simulink model "AC_DCandDC_AC_Conversion"  (R2024a)
settings: Solver=VariableStepAuto  StartTime=0.0  StopTime=5  RelTol=1e-3
undefined symbols (not defined in the file or in its folder): D1, Delta
libraries: spsSeriesRLCBranchLib x6, spsMosfetLib x6, spsVoltageMeasurementLib x5, spsThreePhaseSeriesRLCBranchLib x3, simulink x3, spsCurrentMeasurementLib x2, spsPiSectionLineLib x2, spsThreePhaseSeriesRLCLoadLib x2, spsThreePhaseTransformerTwoWindingsLib x2, spsThreePhaseVIMeasurementLib x2, spsThreePhaseParallelRLCBranchLib x1, spsSawtoothGeneratorLib x1
settings Model: Creator=Esty  LastModifiedBy=Esty

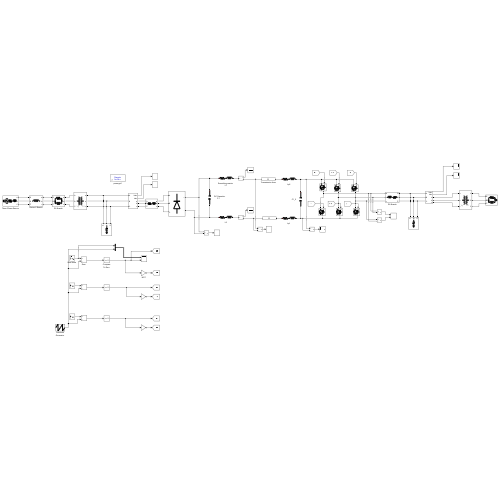
[thumbnail: Simulink's stored preview of the top-level diagram]
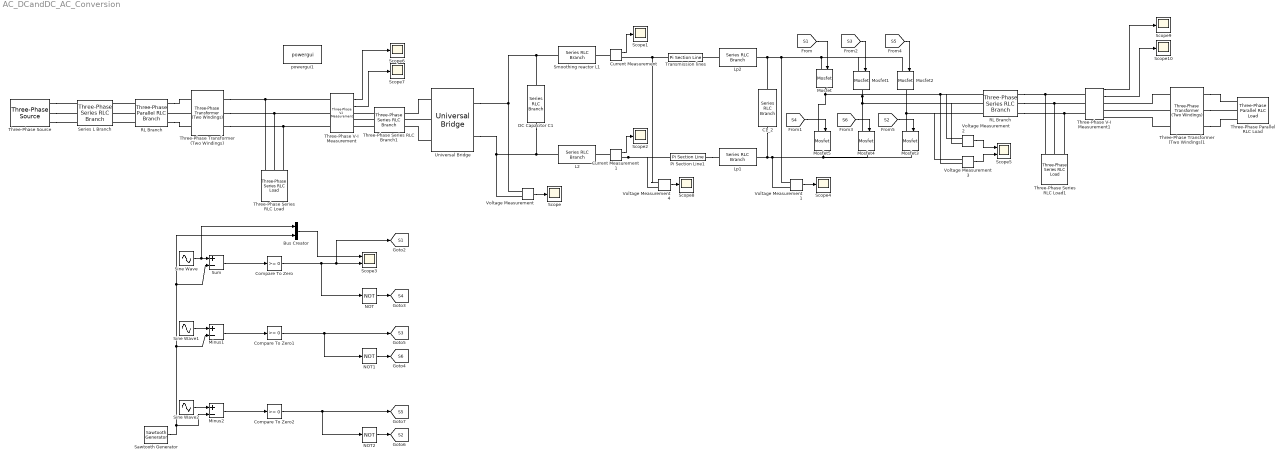
== system AC_DCandDC_AC_Conversion ==
  " RL Branch" : spsThreePhaseSeriesRLCBranchLib/Three-Phase Series RLC Branch  LConnTagsString=A|B|C  RConnTagsString=A|B|C  BranchType=RL  Resistance=0.75  Inductance=0.183  Capacitance=1e-6  Measurements=None
  Bus Creator : BusCreator  Inputs=2
  C1_2 : spsSeriesRLCBranchLib/Series RLC Branch  LConnTagsString=__new0  RConnTagsString=__new0  BranchType=C  Resistance=1  Inductance=1e-3  SetiL0=off  InitialCurrent=0  Capacitance=0.0001  Setx0=off  InitialVoltage=0  Measurements=None
  "Compare To Zero " : simulink/Logic and Bit Operations/Compare To Zero  relop=>=  OutDataTypeStr=boolean
  Compare To Zero1 : simulink/Logic and Bit Operations/Compare To Zero  relop=>=  OutDataTypeStr=boolean
  Compare To Zero2 : simulink/Logic and Bit Operations/Compare To Zero  relop=>=  OutDataTypeStr=boolean
  Current Measurement : spsCurrentMeasurementLib/Current Measurement  PhasorSimulation=off  OutputType=Complex  PSBequivalent=0
  Current Measurement1 : spsCurrentMeasurementLib/Current Measurement  PhasorSimulation=off  OutputType=Complex  PSBequivalent=0
  DC Capacitor C1 : spsSeriesRLCBranchLib/Series RLC Branch  LConnTagsString=__new0  RConnTagsString=__new0  BranchType=C  Resistance=1  Inductance=1e-3  SetiL0=off  InitialCurrent=0  Capacitance=0.005  Setx0=off  InitialVoltage=0  Measurements=None
  L2 : spsSeriesRLCBranchLib/Series RLC Branch  LConnTagsString=__new0  RConnTagsString=__new0  BranchType=RL  Resistance=0.0251  Inductance=1  SetiL0=off  InitialCurrent=0  Capacitance=1e-6  Setx0=off  InitialVoltage=0  Measurements=None
  Lp1 : spsSeriesRLCBranchLib/Series RLC Branch  LConnTagsString=__new0  RConnTagsString=__new0  BranchType=RL  Resistance=0.0251  Inductance=1  SetiL0=off  InitialCurrent=0  Capacitance=1e-6  Setx0=off  InitialVoltage=0  Measurements=None
  Lp2 : spsSeriesRLCBranchLib/Series RLC Branch  LConnTagsString=__new0  RConnTagsString=__new0  BranchType=RL  Resistance=0.0251  Inductance=1  SetiL0=off  InitialCurrent=0  Capacitance=1e-6  Setx0=off  InitialVoltage=0  Measurements=None
  Minus1 : Sum  Inputs=+-
  Minus2 : Sum  Inputs=+-
  Mosfet{,1..5} (6 alike) : spsMosfetLib/Mosfet  Ron=0.1  Lon=0  Rd=0.01  Vfd=0  IC=0  Rs=1e5  Cs=inf  Measurements=off
  "NOT " : Logic  Operator=NOT  IconShape=distinctive  AllPortsSameDT=off  OutDataTypeStr=boolean
  NOT1 : Logic  Operator=NOT  IconShape=distinctive  AllPortsSameDT=off  OutDataTypeStr=boolean
  NOT2 : Logic  Operator=NOT  IconShape=distinctive  AllPortsSameDT=off  OutDataTypeStr=boolean
  Pi Section Line1 : spsPiSectionLineLib/Pi Section Line  LConnTagsString=1  RConnTagsString=1  Phases=1  PiSections=2  Length=75  Frequency=50  Resistance=0.0139  Inductance=0.159e-3  Capacitance=0.23e-6  SpecifyConductance=off  Conductance=0  Measurements=None  Measurements2=None
      settings: LibrarySourceBlock=sps_lib/Power Grid Elements/Pi Section Line
  RL Branch : spsThreePhaseParallelRLCBranchLib/Three-Phase Parallel RLC Branch  LConnTagsString=A|B|C  RConnTagsString=A|B|C  BranchType=RL  Resistance=13.79  Inductance=31.02e-3  Capacitance=1e-6  Measurements=None
  "Sawtooth Generator " : spsSawtoothGeneratorLib/Sawtooth Generator  Freq=5e3  Phase=180  Ts=0
  Scope{,1..2,4,6..10} (9 alike) : Scope
  Scope3 : Scope  NumInputPorts=2
  Scope5 : Scope  NumInputPorts=2
  Series L Branch : spsThreePhaseSeriesRLCBranchLib/Three-Phase Series RLC Branch  LConnTagsString=A|B|C  RConnTagsString=A|B|C  BranchType=L  Resistance=1  Inductance=62.23e-3  Capacitance=1e-6  Measurements=None
  "Sine Wave " : Sin  Frequency=376.99  SampleTime=0
  Sine Wave1 : Sin  Frequency=376.99  Phase=-120*(pi/180)  SampleTime=0
  Sine Wave2 : Sin  Frequency=376.99  Phase=120*(pi/180)  SampleTime=0
  Smoothing reactor L1 : spsSeriesRLCBranchLib/Series RLC Branch  LConnTagsString=__new0  RConnTagsString=__new0  BranchType=RL  Resistance=0.0251  Inductance=1  SetiL0=off  InitialCurrent=0  Capacitance=1e-6  Setx0=off  InitialVoltage=0  Measurements=None
  "Sum " : Sum  Inputs=+-
  Three-Phase Parallel RLC Load : spsThreePhaseParallelRLCLoadLib/Three-Phase Parallel RLC Load  LConnTagsString=A|B|C  Configuration=Y (grounded)  NominalVoltage=230e3  Vabc=[1e3 1e3 1e3]  Vabcp=[1e3 1e3 1e3]  NominalFrequency=50  UnbalancedPower=off  ActivePower=135e3  InductivePower=75e3  CapacitivePower=0  Pabc=[10e3 9e3 11e3]  QLabc=[100 90 110]  QCabc=[100 90 110]  Pabcp=[10e3 9e3 11e3]  QLabcp=[100 90 110]  QCabcp=[100 90 110]  Measurements=None  LoadType=constant Z
  Three-Phase Series RLC Branch1 : spsThreePhaseSeriesRLCBranchLib/Three-Phase Series RLC Branch  LConnTagsString=A|B|C  RConnTagsString=A|B|C  BranchType=RL  Resistance=0.75  Inductance=0.1830  Capacitance=1e-6  Measurements=None
  Three-Phase Series RLC Load : spsThreePhaseSeriesRLCLoadLib/Three-Phase Series RLC Load  LConnTagsString=A|B|C  Configuration=Y (grounded)  NominalVoltage=100e3  Vabc=[1e3 1e3 1e3]  Vabcp=[1e3 1e3 1e3]  NominalFrequency=50  UnbalancedPower=off  ActivePower=0  InductivePower=0  CapacitivePower=200e3  Pabc=[10e3 9e3 11e3]  QLabc=[100 90 110]  QCabc=[100 90 110]  Pabcp=[10e3 9e3 11e3]  QLabcp=[100 90 110]  QCabcp=[100 90 110]  Measurements=None  LoadType=constant Z
  Three-Phase Series RLC Load1 : spsThreePhaseSeriesRLCLoadLib/Three-Phase Series RLC Load  LConnTagsString=A|B|C  Configuration=Y (grounded)  NominalVoltage=100e3  Vabc=[1e3 1e3 1e3]  Vabcp=[1e3 1e3 1e3]  NominalFrequency=50  UnbalancedPower=off  ActivePower=0  InductivePower=0  CapacitivePower=200e3  Pabc=[10e3 9e3 11e3]  QLabc=[100 90 110]  QCabc=[100 90 110]  Pabcp=[10e3 9e3 11e3]  QLabcp=[100 90 110]  QCabcp=[100 90 110]  Measurements=None  LoadType=constant Z
  Three-Phase Transformer (Two Windings) : spsThreePhaseTransformerTwoWindingsLib/Three-Phase Transformer (Two Windings)  Winding1Connection=Yg  Winding2Connection=Delta (D1)  CoreType=Three single-phase transformers  SetSaturation=off  Hysteresis=off  DataFile='hysteresis'  SetInitialFlux=off  Measurements=None  UNITS=pu  NominalPower=[ 200e6 , 50 ]  Winding1=[ 230e3 , 0.0025 , 0.075 ]  Winding2=[ 100e3 , 0.0025 , 0.075 ]  Rm=500  Lm=500  L0=0.5  Saturation=[ 0,0 ; 0.0024,1.2 ; 1.0,1.52 ]  InitialFluxes=[ 0.8 , -0.8 , 0.7 ]  BreakLoop=off  DiscreteSolver=Trapezoidal iterative  DataType=off  TransfoNumber=1
  Three-Phase Transformer (Two Windings)1 : spsThreePhaseTransformerTwoWindingsLib/Three-Phase Transformer (Two Windings)  Winding1Connection=Delta (D1)  Winding2Connection=Yg  CoreType=Three single-phase transformers  SetSaturation=off  Hysteresis=off  DataFile='hysteresis'  SetInitialFlux=off  Measurements=None  UNITS=pu  NominalPower=[ 200e6 , 50 ]  Winding1=[ 230e3*0.88 , 0.0025 , 0.0075 ]  Winding2=[ 100e3 , 0.0025 , 0.075 ]  Rm=500  Lm=500  L0=0.5  Saturation=[ 0,0 ; 0.0024,1.2 ; 1.0,1.52 ]  InitialFluxes=[ 0.8 , -0.8 , 0.7 ]  BreakLoop=off  DiscreteSolver=Trapezoidal iterative  DataType=off  TransfoNumber=1
  Three-Phase V-I Measurement : spsThreePhaseVIMeasurementLib/Three-Phase V-I Measurement  VoltageMeasurement=phase-to-ground  SetLabelV=off  LabelV=Vabc  Vpu=off  VpuLL=off  CurrentMeasurement=yes  SetLabelI=off  LabelI=Iabc  Ipu=off  Pbase=100e6  Vbase=500e3  OutputType=Complex  PhasorSimulation=off  PSBequivalent=0
  Three-Phase V-I Measurement1 : spsThreePhaseVIMeasurementLib/Three-Phase V-I Measurement  VoltageMeasurement=phase-to-ground  SetLabelV=off  LabelV=Vabc  Vpu=off  VpuLL=off  CurrentMeasurement=yes  SetLabelI=off  LabelI=Iabc  Ipu=off  Pbase=100e6  Vbase=500e3  OutputType=Complex  PhasorSimulation=off  PSBequivalent=0
  "Three-Phase Source " : spsThreePhaseSourceLib/Three-Phase Source  InternalConnection=Yg  VoltagePhases=off  Voltage=230e3  PhaseAngle=0  Voltage_phases=[25e3 25e3 25e3]/sqrt(3)  PhaseAngles_phases=[0 -120 +120]  Frequency=50  NonIdealSource=on  SpecifyImpedance=off  Resistance=0.8929  Inductance=16.58e-3  ShortCircuitLevel=100e6  BaseVoltage=25e3  XRratio=7  BusType=swing  Pref=10e3  Qref=0  Prefabc=[10e3, 10e3, 10e3]  Qrefabc=[0, 0, 0]  Qmin=-inf  Qmax=inf
  Transmission lines : spsPiSectionLineLib/Pi Section Line  LConnTagsString=1  RConnTagsString=1  Phases=1  PiSections=2  Length=75  Frequency=50  Resistance=0.0139  Inductance=0.159e-3  Capacitance=0.23e-6  SpecifyConductance=off  Conductance=0  Measurements=None  Measurements2=None
      settings: LibrarySourceBlock=sps_lib/Power Grid Elements/Pi Section Line
  Universal Bridge : spsUniversalBridgeLib/Universal Bridge  Arms=3  SnubberResistance=1e5  SnubberCapacitance=inf  Device=Diodes  Ron=1e-3  Lon=0  ForwardVoltages="[  0  0  ]"  ForwardVoltage=0  GTOparameters=[ 10e-6 , 20e-6 ]  IGBTparameters=[ 1e-6 , 2e-6 ]  Measurements=None  Measurements_2=None  converterType=Rectifier
  Voltage Measurement{,1..4} (5 alike) : spsVoltageMeasurementLib/Voltage Measurement  PhasorSimulation=off  OutputType=Complex  PSBequivalent=0
  powergui1 : sps_lib/powergui  Priority=1  SimulationMode=Discrete  SampleTime=5e-06  frequency=60  Iterations=50  frequencyindice=0  Pbase=100e6  ErrMax=1e-4  UnitsV=kV  UnitsW=MW  buscounter=0  FunctionMessages=off  echomessages=off  EnableUseOfTLC=off  CurrentSourceSwitches=off  DisableSnubberDevices=off  DisableRonSwitches=off  DisableVfSwitches=off  DisplayEquations=off  AutomaticDiscreteSolvers=off  SolverType=Tustin/Backward Euler (TBE)  Interpol=off  ExternalGateDelay=off  methode=off  Ts=100  x0status=blocks  SPID=on  SwTol=0  HookPort=off  NonlinearTolerance=1e-4  nMaxIteration=100  ContinueOnMaxIteration=off  RestoreLinks=warning  ResistiveCurrentMeasurement=off  Frange=[0:2:500]  Ylog=off  Xlog=on  ShowGrid=off  save=off  variable=ZData  structure=0  ZoomFFT=off  StartTime=0.0  cycles=1  DisplayStyle=1  fundamental=60  FreqAxis=off  MaxFrequency=1000  frequencyindicesteady=1  RmsSteady=1  display=off
  tag scope: S1=global, S2=global, S3=global, S4=global, S5=global, S6=global
  wires:
  Voltage Measurement/1 -> Scope/1
  Current Measurement/1 -> Scope1/1
  Current Measurement1/1 -> Scope2/1
  [S4] -> Mosfet5/1
  [S3] -> Mosfet1/1
  [S5] -> Mosfet2/1
  [S2] -> Mosfet3/1
  [S6] -> Mosfet4/1
  Minus2/1 -> Compare To Zero2/1
  "Sum "/1 -> "Compare To Zero "/1
  "Sine Wave "/1 -> Bus Creator/1, "Sum "/1
  Compare To Zero1/1 -> [S3], NOT1/1
  Bus Creator/1 -> Scope3/1
  "NOT "/1 -> [S4]
  Compare To Zero2/1 -> [S5], NOT2/1
  Sine Wave2/1 -> Minus2/1
  "Sawtooth Generator "/1 -> Bus Creator/2, "Sum "/2, Minus1/2, Minus2/2
  NOT2/1 -> [S2]
  Minus1/1 -> Compare To Zero1/1
  "Compare To Zero "/1 -> "NOT "/1, [S1], Scope3/2
  Sine Wave1/1 -> Minus1/1
  NOT1/1 -> [S6]
  [S1] -> Mosfet/1
  Voltage Measurement1/1 -> Scope4/1
  Voltage Measurement2/1 -> Scope5/1
  Voltage Measurement3/1 -> Scope5/2
  Three-Phase V-I Measurement/1 -> Scope6/1
  Three-Phase V-I Measurement/2 -> Scope7/1
  Voltage Measurement4/1 -> Scope8/1
  Three-Phase V-I Measurement1/1 -> Scope9/1
  Three-Phase V-I Measurement1/2 -> Scope10/1
  connections:
  "Three-Phase Source "/RConn1 -- Series L Branch/LConn1
  "Three-Phase Source "/RConn2 -- Series L Branch/LConn2
  "Three-Phase Source "/RConn3 -- Series L Branch/LConn3
  RL Branch/LConn1 -- Series L Branch/RConn1
  RL Branch/LConn2 -- Series L Branch/RConn2
  RL Branch/LConn3 -- Series L Branch/RConn3
  Three-Phase Transformer (Two Windings)/LConn2 -- RL Branch/RConn2
  RL Branch/RConn1 -- Three-Phase Transformer (Two Windings)/LConn1
  RL Branch/RConn3 -- Three-Phase Transformer (Two Windings)/LConn3
  Three-Phase Transformer (Two Windings)/RConn1 -- Three-Phase Series RLC Load/LConn1 -- Three-Phase V-I Measurement/LConn1
  Three-Phase Transformer (Two Windings)/RConn2 -- Three-Phase V-I Measurement/LConn2 -- Three-Phase Series RLC Load/LConn2
  Three-Phase Transformer (Two Windings)/RConn3 -- Three-Phase V-I Measurement/LConn3 -- Three-Phase Series RLC Load/LConn3
  Universal Bridge/LConn1 -- Three-Phase Series RLC Branch1/RConn1
  Universal Bridge/LConn2 -- Three-Phase Series RLC Branch1/RConn2
  Universal Bridge/LConn3 -- Three-Phase Series RLC Branch1/RConn3
  Universal Bridge/RConn1 -- DC Capacitor C1/LConn1 -- Smoothing reactor L1/LConn1 -- Voltage Measurement/LConn1
  Current Measurement1/LConn1 -- L2/RConn1
  Current Measurement/LConn1 -- Smoothing reactor L1/RConn1
  Universal Bridge/RConn2 -- Voltage Measurement/LConn2 -- DC Capacitor C1/RConn1 -- L2/LConn1
  Transmission lines/LConn1 -- Voltage Measurement4/LConn1 -- Current Measurement/RConn1
  Current Measurement1/RConn1 -- Pi Section Line1/LConn1 -- Voltage Measurement4/LConn2
  Pi Section Line1/RConn1 -- Lp1/LConn1
  Lp2/LConn1 -- Transmission lines/RConn1
  Mosfet2/LConn1 -- Mosfet1/LConn1 -- Mosfet/LConn1 -- Voltage Measurement1/LConn1 -- Lp2/RConn1 -- C1_2/LConn1
  Mosfet3/RConn1 -- Mosfet4/RConn1 -- Voltage Measurement1/LConn2 -- C1_2/RConn1 -- Lp1/RConn1 -- Mosfet5/RConn1
  Mosfet3/LConn1 -- Mosfet2/RConn1 -- " RL Branch"/RConn3 -- Voltage Measurement3/LConn1
  Mosfet5/LConn1 -- " RL Branch"/RConn1 -- Voltage Measurement2/LConn1 -- Voltage Measurement3/LConn2 -- Mosfet/RConn1
  Mosfet1/RConn1 -- " RL Branch"/RConn2 -- Voltage Measurement2/LConn2 -- Mosfet4/LConn1
  Three-Phase Series RLC Load1/LConn2 -- " RL Branch"/LConn2 -- Three-Phase V-I Measurement1/LConn2
  Three-Phase Series RLC Load1/LConn1 -- " RL Branch"/LConn1 -- Three-Phase V-I Measurement1/LConn1
  Three-Phase Series RLC Load1/LConn3 -- " RL Branch"/LConn3 -- Three-Phase V-I Measurement1/LConn3
  Three-Phase Transformer (Two Windings)1/LConn1 -- Three-Phase Parallel RLC Load/LConn1
  Three-Phase Transformer (Two Windings)1/LConn2 -- Three-Phase Parallel RLC Load/LConn2
  Three-Phase Transformer (Two Windings)1/LConn3 -- Three-Phase Parallel RLC Load/LConn3
  Three-Phase Series RLC Branch1/LConn1 -- Three-Phase V-I Measurement/RConn1
  Three-Phase Series RLC Branch1/LConn2 -- Three-Phase V-I Measurement/RConn2
  Three-Phase Series RLC Branch1/LConn3 -- Three-Phase V-I Measurement/RConn3
  Three-Phase Transformer (Two Windings)1/RConn1 -- Three-Phase V-I Measurement1/RConn1
  Three-Phase Transformer (Two Windings)1/RConn2 -- Three-Phase V-I Measurement1/RConn2
  Three-Phase Transformer (Two Windings)1/RConn3 -- Three-Phase V-I Measurement1/RConn3
